simulink library "inp"  (R2021b)
settings: Solver=VariableStepAuto  StartTime=0.0  StopTime=10.0  RelTol=1e-3
undefined symbols (not defined in the file): C_TASK_5MS_S, FALSE, KINP_AcoreReadyToSlp_flg_ovrdflg, KINP_AcoreReadyToSlp_flg_ovrdval, KINP_AllowMovThd_OTA_enum_ovrdflg, KINP_AllowMovThd_OTA_enum_ovrdval, KINP_APSAngleTarget_Deg_ovrdflg, KINP_APSAngleTarget_Deg_ovrdval, KINP_APSDecReq_mps2_ovrdflg, KINP_APSDecReq_mps2_ovrdval, KINP_APSDecReqA_flg_ovrdflg, KINP_APSDecReqA_flg_ovrdval, KINP_APSDFLL_cm_ovrdflg, KINP_APSDFLL_cm_ovrdval, KINP_APSDFLR_cm_ovrdflg, KINP_APSDFLR_cm_ovrdval, KINP_APSDRLL_cm_ovrdflg, KINP_APSDRLL_cm_ovrdval, KINP_APSDRLR_cm_ovrdflg, KINP_APSDRLR_cm_ovrdval, KINP_APSExitCondition_enum_ovrdflg, KINP_APSExitCondition_enum_ovrdval, KINP_APSHWVer_enum_ovrdflg, KINP_APSHWVer_enum_ovrdval, KINP_APSProgressPCT_pct_ovrdflg, KINP_APSProgressPCT_pct_ovrdval, KINP_APSReq_enum_ovrdflg, KINP_APSReq_enum_ovrdval, KINP_APSRQDisplay_enum_ovrdflg, KINP_APSRQDisplay_enum_ovrdval, KINP_APSRqEPASCtrl_flg_ovrdflg, KINP_APSRqEPASCtrl_flg_ovrdval, KINP_APSShiftPosnReq_enum_ovrdval, KINP_APSShiftPosnReq_enum_ovrflg, KINP_APSSpeedCMD_kph_ovrdval, KINP_APSSpeedCMD_kph_ovrflg, KINP_APSStaSystem_enum_ovrdflg, KINP_APSStaSystem_enum_ovrdval, KINP_APSSWVer_enum_ovrdflg, KINP_APSSWVer_enum_ovrdval, KINP_APSVMCReqA_flg_ovrdval, KINP_APSVMCReqA_flg_ovrflg, KINP_APSVRqEPASCtrl_flg_ovrdflg, KINP_APSVRqEPASCtrl_flg_ovrdval, KINP_AuxBattVolmV_mV_ovrdflg, KINP_AuxBattVolmV_mV_ovrdval, KINP_CAASSta_enum_ovrdflg, KINP_CAASSta_enum_ovrdval, KINP_CAASVMCReqA_flg_ovrdval, KINP_CAASVMCReqA_flg_ovrflg, KINP_Chime_enum_ovrdflg, KINP_Chime_enum_ovrdval, KINP_ClearDTCcmd_flg_ovrdflg, KINP_ClearDTCcmd_flg_ovrdval, KINP_EvccAplusPwrUpReq_flg_ovrdflg, KINP_EvccAplusPwrUpReq_flg_ovrdval, KINP_LFID_raw_ovrdval, KINP_LFID_raw_ovrflg, KINP_LRID_raw_ovrdval, KINP_MemOffsetAccX_raw16_ovrdflg ... (+118)
libraries: FVT_lib x942, hcu_lib x1
(part 20 of 31)

== system inp/INP/CAN3/SignalCheck/MCU_B_R1 ==
  BHAL_outputs : Inport
  inp_CanValid_bus : Inport  Port=2
  MCUWarnR : FVT_lib/inp/can_signal_template  SystemSampleTime=-1  VariantActivationTime=update diagram  Latency=0  AutoFrameSizeCalculation=off
      link override defval: Value=KINP_MCUWarnR_enum_defval
      link override ovrdflg: Value=KINP_MCUWarnR_enum_ovrdflg
      link override ovrdval: Value=KINP_MCUWarnR_enum_ovrdval
  RrActvDmpDisabSta : FVT_lib/inp/can_signal_template  SystemSampleTime=-1  VariantActivationTime=update diagram  Latency=0  AutoFrameSizeCalculation=off
      link override defval: Value=KINP_RrActvDmpDisabSta_flg_defval
      link override ovrdflg: Value=KINP_RrActvDmpDisabSta_flg_ovrdflg
      link override ovrdval: Value=KINP_RrActvDmpDisabSta_flg_ovrdval
  RrEDUDrtSta : FVT_lib/inp/can_signal_template  SystemSampleTime=-1  VariantActivationTime=update diagram  Latency=0  AutoFrameSizeCalculation=off
      link override defval: Value=KINP_RrEDUDrtSta_flg_defval
      link override ovrdflg: Value=KINP_RrEDUDrtSta_flg_ovrdflg
      link override ovrdval: Value=KINP_RrEDUDrtSta_flg_ovrdval
  RrEDUOpratingSta : FVT_lib/inp/can_signal_template  SystemSampleTime=-1  VariantActivationTime=update diagram  Latency=0  AutoFrameSizeCalculation=off
      link override defval: Value=KINP_RrEDUOpratingSta_flg_defval
      link override ovrdflg: Value=KINP_RrEDUOpratingSta_flg_ovrdflg
      link override ovrdval: Value=KINP_RrEDUOpratingSta_flg_ovrdval
  RrEDURealTMTq : FVT_lib/inp/can_signal_template  SystemSampleTime=-1  VariantActivationTime=update diagram  Latency=0  AutoFrameSizeCalculation=off
      link override defval: Value=KINP_RrEDURealTMTq_Nm_defval
      link override ovrdflg: Value=KINP_RrEDURealTMTq_Nm_ovrdflg
      link override ovrdval: Value=KINP_RrEDURealTMTq_Nm_ovrdval
  RrEDURotateDirction : FVT_lib/inp/can_signal_template  SystemSampleTime=-1  VariantActivationTime=update diagram  Latency=0  AutoFrameSizeCalculation=off
      link override defval: Value=KINP_RrEDURotateDirction_enum_defval
      link override ovrdflg: Value=KINP_RrEDURotateDirction_enum_ovrdflg
      link override ovrdval: Value=KINP_RrEDURotateDirction_enum_ovrdval
  RrEDUTqReqFbk : FVT_lib/inp/can_signal_template  SystemSampleTime=-1  VariantActivationTime=update diagram  Latency=0  AutoFrameSizeCalculation=off
      link override defval: Value=KINP_RrEDUTqReqFbk_Nm_defval
      link override ovrdflg: Value=KINP_RrEDUTqReqFbk_Nm_ovrdflg
      link override ovrdval: Value=KINP_RrEDUTqReqFbk_Nm_ovrdval
  RrMCUBAT : FVT_lib/inp/can_signal_template  SystemSampleTime=-1  VariantActivationTime=update diagram  Latency=0  AutoFrameSizeCalculation=off
      link override defval: Value=KINP_RrMCUBAT_V_defval
      link override ovrdflg: Value=KINP_RrMCUBAT_V_ovrdflg
      link override ovrdval: Value=KINP_RrMCUBAT_V_ovrdval
  RrMCUDCBusCurr : FVT_lib/inp/can_signal_template  SystemSampleTime=-1  VariantActivationTime=update diagram  Latency=0  AutoFrameSizeCalculation=off
      link override defval: Value=KINP_RrMCUDCBusCurr_A_defval
      link override ovrdflg: Value=KINP_RrMCUDCBusCurr_A_ovrdflg
      link override ovrdval: Value=KINP_RrMCUDCBusCurr_A_ovrdval
  RrMCUDCBusVolt : FVT_lib/inp/can_signal_template  SystemSampleTime=-1  VariantActivationTime=update diagram  Latency=0  AutoFrameSizeCalculation=off
      link override defval: Value=KINP_RrMCUDCBusVolt_V_defval
      link override ovrdflg: Value=KINP_RrMCUDCBusVolt_V_ovrdflg
      link override ovrdval: Value=KINP_RrMCUDCBusVolt_V_ovrdval
  RrMCUDischrgSta : FVT_lib/inp/can_signal_template  SystemSampleTime=-1  VariantActivationTime=update diagram  Latency=0  AutoFrameSizeCalculation=off
      link override defval: Value=KINP_RrMCUDischrgSta_flg_defval
      link override ovrdflg: Value=KINP_RrMCUDischrgSta_flg_ovrdflg
      link override ovrdval: Value=KINP_RrMCUDischrgSta_flg_ovrdval
  RrMCUEnaSta : FVT_lib/inp/can_signal_template  SystemSampleTime=-1  VariantActivationTime=update diagram  Latency=0  AutoFrameSizeCalculation=off
      link override defval: Value=KINP_RrMCUEnaSta_flg_defval
      link override ovrdflg: Value=KINP_RrMCUEnaSta_flg_ovrdflg
      link override ovrdval: Value=KINP_RrMCUEnaSta_flg_ovrdval
  RrMCUErr : FVT_lib/inp/can_signal_template  SystemSampleTime=-1  VariantActivationTime=update diagram  Latency=0  AutoFrameSizeCalculation=off
      link override defval: Value=KINP_RrMCUErr_enum_defval
      link override ovrdflg: Value=KINP_RrMCUErr_enum_ovrdflg
      link override ovrdval: Value=KINP_RrMCUErr_enum_ovrdval
  RrMCUIGNsta : FVT_lib/inp/can_signal_template  SystemSampleTime=-1  VariantActivationTime=update diagram  Latency=0  AutoFrameSizeCalculation=off
      link override defval: Value=KINP_RrMCUIGNsta_flg_defval
      link override ovrdflg: Value=KINP_RrMCUIGNsta_flg_ovrdflg
      link override ovrdval: Value=KINP_RrMCUIGNsta_flg_ovrdval
  RrMCUReady : FVT_lib/inp/can_signal_template  SystemSampleTime=-1  VariantActivationTime=update diagram  Latency=0  AutoFrameSizeCalculation=off
      link override defval: Value=KINP_RrMCUReady_flg_defval
      link override ovrdflg: Value=KINP_RrMCUReady_flg_ovrdflg
      link override ovrdval: Value=KINP_RrMCUReady_flg_ovrdval
  RrMCUReady4Pre : FVT_lib/inp/can_signal_template  SystemSampleTime=-1  VariantActivationTime=update diagram  Latency=0  AutoFrameSizeCalculation=off
      link override defval: Value=KINP_RrMCUReady4Pre_flg_defval
      link override ovrdflg: Value=KINP_RrMCUReady4Pre_flg_ovrdflg
      link override ovrdval: Value=KINP_RrMCUReady4Pre_flg_ovrdval
  RrMCUSysSta : FVT_lib/inp/can_signal_template  SystemSampleTime=-1  VariantActivationTime=update diagram  Latency=0  AutoFrameSizeCalculation=off
      link override defval: Value=KINP_RrMCUSysSta_enum_defval
      link override ovrdflg: Value=KINP_RrMCUSysSta_enum_ovrdflg
      link override ovrdval: Value=KINP_RrMCUSysSta_enum_ovrdval
  RrMCUTemp : FVT_lib/inp/can_signal_template  SystemSampleTime=-1  VariantActivationTime=update diagram  Latency=0  AutoFrameSizeCalculation=off
      link override defval: Value=KINP_RrMCUTemp_C_defval
      link override ovrdflg: Value=KINP_RrMCUTemp_C_ovrdflg
      link override ovrdval: Value=KINP_RrMCUTemp_C_ovrdval
  RrMotorAvailTq : FVT_lib/inp/can_signal_template  SystemSampleTime=-1  VariantActivationTime=update diagram  Latency=0  AutoFrameSizeCalculation=off
      link override defval: Value=KINP_RrMotorAvailTq_Nm_defval
      link override ovrdflg: Value=KINP_RrMotorAvailTq_Nm_ovrdflg
      link override ovrdval: Value=KINP_RrMotorAvailTq_Nm_ovrdval
  RrRegenAvailTq : FVT_lib/inp/can_signal_template  SystemSampleTime=-1  VariantActivationTime=update diagram  Latency=0  AutoFrameSizeCalculation=off
      link override defval: Value=KINP_RrRegenAvailTq_Nm_defval
      link override ovrdflg: Value=KINP_RrRegenAvailTq_Nm_ovrdflg
      link override ovrdval: Value=KINP_RrRegenAvailTq_Nm_ovrdval
  RrTMSpd : FVT_lib/inp/can_signal_template  SystemSampleTime=-1  VariantActivationTime=update diagram  Latency=0  AutoFrameSizeCalculation=off
      link override defval: Value=KINP_RrTMSpd_rpm_defval
      link override ovrdflg: Value=KINP_RrTMSpd_rpm_ovrdflg
      link override ovrdval: Value=KINP_RrTMSpd_rpm_ovrdval
  RrTMTemp : FVT_lib/inp/can_signal_template  SystemSampleTime=-1  VariantActivationTime=update diagram  Latency=0  AutoFrameSizeCalculation=off
      link override defval: Value=KINP_RrTMTemp_C_defval
      link override ovrdflg: Value=KINP_RrTMTemp_C_ovrdflg
      link override ovrdval: Value=KINP_RrTMTemp_C_ovrdval
  RrTMid : FVT_lib/inp/can_signal_template  SystemSampleTime=-1  VariantActivationTime=update diagram  Latency=0  AutoFrameSizeCalculation=off
      link override defval: Value=KINP_RrTMid_A_defval
      link override ovrdflg: Value=KINP_RrTMid_A_ovrdflg
      link override ovrdval: Value=KINP_RrTMid_A_ovrdval
  RrTMiq : FVT_lib/inp/can_signal_template  SystemSampleTime=-1  VariantActivationTime=update diagram  Latency=0  AutoFrameSizeCalculation=off
      link override defval: Value=KINP_RrTMiq_A_defval
      link override ovrdflg: Value=KINP_RrTMiq_A_ovrdflg
      link override ovrdval: Value=KINP_RrTMiq_A_ovrdval
  Terminator_{1..24} (24 alike) : Terminator
  True_VHAL_MCUWarnR_enum : Constant  Value=TRUE  OutDataTypeStr=boolean
  True_VHAL_RrActvDmpDisabSta_flg : Constant  Value=TRUE  OutDataTypeStr=boolean
  True_VHAL_RrEDUDrtSta_flg : Constant  Value=TRUE  OutDataTypeStr=boolean
  True_VHAL_RrEDUOpratingSta_flg : Constant  Value=TRUE  OutDataTypeStr=boolean
  True_VHAL_RrEDURealTMTq_Nm : Constant  Value=TRUE  OutDataTypeStr=boolean
  True_VHAL_RrEDURotateDirction_enum : Constant  Value=TRUE  OutDataTypeStr=boolean
  True_VHAL_RrEDUTqReqFbk_Nm : Constant  Value=TRUE  OutDataTypeStr=boolean
  True_VHAL_RrMCUBAT_V : Constant  Value=TRUE  OutDataTypeStr=boolean
  True_VHAL_RrMCUDCBusCurr_A : Constant  Value=TRUE  OutDataTypeStr=boolean
  True_VHAL_RrMCUDCBusVolt_V : Constant  Value=TRUE  OutDataTypeStr=boolean
  True_VHAL_RrMCUDischrgSta_flg : Constant  Value=TRUE  OutDataTypeStr=boolean
  True_VHAL_RrMCUEnaSta_flg : Constant  Value=TRUE  OutDataTypeStr=boolean
  True_VHAL_RrMCUErr_enum : Constant  Value=TRUE  OutDataTypeStr=boolean
  True_VHAL_RrMCUIGNsta_flg : Constant  Value=TRUE  OutDataTypeStr=boolean
  True_VHAL_RrMCUReady4Pre_flg : Constant  Value=TRUE  OutDataTypeStr=boolean
  True_VHAL_RrMCUReady_flg : Constant  Value=TRUE  OutDataTypeStr=boolean
  True_VHAL_RrMCUSysSta_enum : Constant  Value=TRUE  OutDataTypeStr=boolean
  True_VHAL_RrMCUTemp_C : Constant  Value=TRUE  OutDataTypeStr=boolean
  True_VHAL_RrMotorAvailTq_Nm : Constant  Value=TRUE  OutDataTypeStr=boolean
  True_VHAL_RrRegenAvailTq_Nm : Constant  Value=TRUE  OutDataTypeStr=boolean
  True_VHAL_RrTMSpd_rpm : Constant  Value=TRUE  OutDataTypeStr=boolean
  True_VHAL_RrTMTemp_C : Constant  Value=TRUE  OutDataTypeStr=boolean
  True_VHAL_RrTMid_A : Constant  Value=TRUE  OutDataTypeStr=boolean
  True_VHAL_RrTMiq_A : Constant  Value=TRUE  OutDataTypeStr=boolean
  slr1_{1..24} (24 alike) : BusSelector  OutputSignals=VINP_CANMsgValidMCUBR1_flg
  slr_VHAL_MCUWarnR_enum : BusSelector  OutputSignals=VHAL_MCUWarnR_enum
  slr_VHAL_RrActvDmpDisabSta_flg : BusSelector  OutputSignals=VHAL_RrActvDmpDisabSta_flg
  slr_VHAL_RrEDUDrtSta_flg : BusSelector  OutputSignals=VHAL_RrEDUDrtSta_flg
  slr_VHAL_RrEDUOpratingSta_flg : BusSelector  OutputSignals=VHAL_RrEDUOpratingSta_flg
  slr_VHAL_RrEDURealTMTq_Nm : BusSelector  OutputSignals=VHAL_RrEDURealTMTq_Nm
  slr_VHAL_RrEDURotateDirction_enum : BusSelector  OutputSignals=VHAL_RrEDURotateDirction_enum
  slr_VHAL_RrEDUTqReqFbk_Nm : BusSelector  OutputSignals=VHAL_RrEDUTqReqFbk_Nm
  slr_VHAL_RrMCUBAT_V : BusSelector  OutputSignals=VHAL_RrMCUBAT_V
  slr_VHAL_RrMCUDCBusCurr_A : BusSelector  OutputSignals=VHAL_RrMCUDCBusCurr_A
  slr_VHAL_RrMCUDCBusVolt_V : BusSelector  OutputSignals=VHAL_RrMCUDCBusVolt_V
  slr_VHAL_RrMCUDischrgSta_flg : BusSelector  OutputSignals=VHAL_RrMCUDischrgSta_flg
  slr_VHAL_RrMCUEnaSta_flg : BusSelector  OutputSignals=VHAL_RrMCUEnaSta_flg
  slr_VHAL_RrMCUErr_enum : BusSelector  OutputSignals=VHAL_RrMCUErr_enum
  slr_VHAL_RrMCUIGNsta_flg : BusSelector  OutputSignals=VHAL_RrMCUIGNsta_flg
  slr_VHAL_RrMCUReady4Pre_flg : BusSelector  OutputSignals=VHAL_RrMCUReady4Pre_flg
  slr_VHAL_RrMCUReady_flg : BusSelector  OutputSignals=VHAL_RrMCUReady_flg
  slr_VHAL_RrMCUSysSta_enum : BusSelector  OutputSignals=VHAL_RrMCUSysSta_enum
  slr_VHAL_RrMCUTemp_C : BusSelector  OutputSignals=VHAL_RrMCUTemp_C
  slr_VHAL_RrMotorAvailTq_Nm : BusSelector  OutputSignals=VHAL_RrMotorAvailTq_Nm
  slr_VHAL_RrRegenAvailTq_Nm : BusSelector  OutputSignals=VHAL_RrRegenAvailTq_Nm
  slr_VHAL_RrTMSpd_rpm : BusSelector  OutputSignals=VHAL_RrTMSpd_rpm
  slr_VHAL_RrTMTemp_C : BusSelector  OutputSignals=VHAL_RrTMTemp_C
  slr_VHAL_RrTMid_A : BusSelector  OutputSignals=VHAL_RrTMid_A
  slr_VHAL_RrTMiq_A : BusSelector  OutputSignals=VHAL_RrTMiq_A
  VINP_MCUWarnR_enum : Outport
  VINP_RrActvDmpDisabSta_flg : Outport  Port=2
  VINP_RrEDUDrtSta_flg : Outport  Port=3
  VINP_RrEDUOpratingSta_flg : Outport  Port=4
  VINP_RrEDURealTMTq_Nm : Outport  Port=5
  VINP_RrEDURotateDirction_enum : Outport  Port=6
  VINP_RrEDUTqReqFbk_Nm : Outport  Port=7
  VINP_RrMCUBAT_V : Outport  Port=8
  VINP_RrMCUDCBusCurr_A : Outport  Port=9
  VINP_RrMCUDCBusVolt_V : Outport  Port=10
  VINP_RrMCUDischrgSta_flg : Outport  Port=11
  VINP_RrMCUEnaSta_flg : Outport  Port=12
  VINP_RrMCUErr_enum : Outport  Port=13
  VINP_RrMCUIGNsta_flg : Outport  Port=14
  VINP_RrMCUReady_flg : Outport  Port=15
  VINP_RrMCUReady4Pre_flg : Outport  Port=16
  VINP_RrMCUSysSta_enum : Outport  Port=17
  VINP_RrMCUTemp_C : Outport  Port=18
  VINP_RrMotorAvailTq_Nm : Outport  Port=19
  VINP_RrRegenAvailTq_Nm : Outport  Port=20
  VINP_RrTMSpd_rpm : Outport  Port=21
  VINP_RrTMTemp_C : Outport  Port=22
  VINP_RrTMid_A : Outport  Port=23
  VINP_RrTMiq_A : Outport  Port=24
  wires:
  BHAL_outputs/1 -> [BHAL_outputs]
  inp_CanValid_bus/1 -> [inp_CanValid_bus]
  [BHAL_outputs] -> slr_VHAL_MCUWarnR_enum/1
  slr_VHAL_MCUWarnR_enum/1 -> MCUWarnR/1  "<VHAL_MCUWarnR_enum>"
  True_VHAL_MCUWarnR_enum/1 -> MCUWarnR/2
  [inp_CanValid_bus] -> slr1_1/1
  slr1_1/1 -> MCUWarnR/3  "<VINP_CANMsgValidMCUBR1_flg>"
  MCUWarnR/1 -> VINP_MCUWarnR_enum/1  "VINP_MCUWarnR_enum"
  MCUWarnR/2 -> Terminator_1/1
  [BHAL_outputs] -> slr_VHAL_RrActvDmpDisabSta_flg/1
  slr_VHAL_RrActvDmpDisabSta_flg/1 -> RrActvDmpDisabSta/1  "<VHAL_RrActvDmpDisabSta_flg>"
  True_VHAL_RrActvDmpDisabSta_flg/1 -> RrActvDmpDisabSta/2
  [inp_CanValid_bus] -> slr1_2/1
  slr1_2/1 -> RrActvDmpDisabSta/3  "<VINP_CANMsgValidMCUBR1_flg>"
  RrActvDmpDisabSta/1 -> VINP_RrActvDmpDisabSta_flg/1  "VINP_RrActvDmpDisabSta_flg"
  RrActvDmpDisabSta/2 -> Terminator_2/1
  [BHAL_outputs] -> slr_VHAL_RrEDUDrtSta_flg/1
  slr_VHAL_RrEDUDrtSta_flg/1 -> RrEDUDrtSta/1  "<VHAL_RrEDUDrtSta_flg>"
  True_VHAL_RrEDUDrtSta_flg/1 -> RrEDUDrtSta/2
  [inp_CanValid_bus] -> slr1_3/1
  slr1_3/1 -> RrEDUDrtSta/3  "<VINP_CANMsgValidMCUBR1_flg>"
  RrEDUDrtSta/1 -> VINP_RrEDUDrtSta_flg/1  "VINP_RrEDUDrtSta_flg"
  RrEDUDrtSta/2 -> Terminator_3/1
  [BHAL_outputs] -> slr_VHAL_RrEDUOpratingSta_flg/1
  slr_VHAL_RrEDUOpratingSta_flg/1 -> RrEDUOpratingSta/1  "<VHAL_RrEDUOpratingSta_flg>"
  True_VHAL_RrEDUOpratingSta_flg/1 -> RrEDUOpratingSta/2
  [inp_CanValid_bus] -> slr1_4/1
  slr1_4/1 -> RrEDUOpratingSta/3  "<VINP_CANMsgValidMCUBR1_flg>"
  RrEDUOpratingSta/1 -> VINP_RrEDUOpratingSta_flg/1  "VINP_RrEDUOpratingSta_flg"
  RrEDUOpratingSta/2 -> Terminator_4/1
  [BHAL_outputs] -> slr_VHAL_RrEDURealTMTq_Nm/1
  slr_VHAL_RrEDURealTMTq_Nm/1 -> RrEDURealTMTq/1  "<VHAL_RrEDURealTMTq_Nm>"
  True_VHAL_RrEDURealTMTq_Nm/1 -> RrEDURealTMTq/2
  [inp_CanValid_bus] -> slr1_5/1
  slr1_5/1 -> RrEDURealTMTq/3  "<VINP_CANMsgValidMCUBR1_flg>"
  RrEDURealTMTq/1 -> VINP_RrEDURealTMTq_Nm/1  "VINP_RrEDURealTMTq_Nm"
  RrEDURealTMTq/2 -> Terminator_5/1
  [BHAL_outputs] -> slr_VHAL_RrEDURotateDirction_enum/1
  slr_VHAL_RrEDURotateDirction_enum/1 -> RrEDURotateDirction/1  "<VHAL_RrEDURotateDirction_enum>"
  True_VHAL_RrEDURotateDirction_enum/1 -> RrEDURotateDirction/2
  [inp_CanValid_bus] -> slr1_6/1
  slr1_6/1 -> RrEDURotateDirction/3  "<VINP_CANMsgValidMCUBR1_flg>"
  RrEDURotateDirction/1 -> VINP_RrEDURotateDirction_enum/1  "VINP_RrEDURotateDirction_enum"
  RrEDURotateDirction/2 -> Terminator_6/1
  [BHAL_outputs] -> slr_VHAL_RrEDUTqReqFbk_Nm/1
  slr_VHAL_RrEDUTqReqFbk_Nm/1 -> RrEDUTqReqFbk/1  "<VHAL_RrEDUTqReqFbk_Nm>"
  True_VHAL_RrEDUTqReqFbk_Nm/1 -> RrEDUTqReqFbk/2
  [inp_CanValid_bus] -> slr1_7/1
  slr1_7/1 -> RrEDUTqReqFbk/3  "<VINP_CANMsgValidMCUBR1_flg>"
  RrEDUTqReqFbk/1 -> VINP_RrEDUTqReqFbk_Nm/1  "VINP_RrEDUTqReqFbk_Nm"
  RrEDUTqReqFbk/2 -> Terminator_7/1
  [BHAL_outputs] -> slr_VHAL_RrMCUBAT_V/1
  slr_VHAL_RrMCUBAT_V/1 -> RrMCUBAT/1  "<VHAL_RrMCUBAT_V>"
  True_VHAL_RrMCUBAT_V/1 -> RrMCUBAT/2
  [inp_CanValid_bus] -> slr1_8/1
  slr1_8/1 -> RrMCUBAT/3  "<VINP_CANMsgValidMCUBR1_flg>"
  RrMCUBAT/1 -> VINP_RrMCUBAT_V/1  "VINP_RrMCUBAT_V"
  RrMCUBAT/2 -> Terminator_8/1
  [BHAL_outputs] -> slr_VHAL_RrMCUDCBusCurr_A/1
  slr_VHAL_RrMCUDCBusCurr_A/1 -> RrMCUDCBusCurr/1  "<VHAL_RrMCUDCBusCurr_A>"
  True_VHAL_RrMCUDCBusCurr_A/1 -> RrMCUDCBusCurr/2
  [inp_CanValid_bus] -> slr1_9/1
  slr1_9/1 -> RrMCUDCBusCurr/3  "<VINP_CANMsgValidMCUBR1_flg>"
  RrMCUDCBusCurr/1 -> VINP_RrMCUDCBusCurr_A/1  "VINP_RrMCUDCBusCurr_A"
  RrMCUDCBusCurr/2 -> Terminator_9/1
  [BHAL_outputs] -> slr_VHAL_RrMCUDCBusVolt_V/1
  slr_VHAL_RrMCUDCBusVolt_V/1 -> RrMCUDCBusVolt/1  "<VHAL_RrMCUDCBusVolt_V>"
  True_VHAL_RrMCUDCBusVolt_V/1 -> RrMCUDCBusVolt/2
  [inp_CanValid_bus] -> slr1_10/1
  slr1_10/1 -> RrMCUDCBusVolt/3  "<VINP_CANMsgValidMCUBR1_flg>"
  RrMCUDCBusVolt/1 -> VINP_RrMCUDCBusVolt_V/1  "VINP_RrMCUDCBusVolt_V"
  RrMCUDCBusVolt/2 -> Terminator_10/1
  [BHAL_outputs] -> slr_VHAL_RrMCUDischrgSta_flg/1
  slr_VHAL_RrMCUDischrgSta_flg/1 -> RrMCUDischrgSta/1  "<VHAL_RrMCUDischrgSta_flg>"
  True_VHAL_RrMCUDischrgSta_flg/1 -> RrMCUDischrgSta/2
  [inp_CanValid_bus] -> slr1_11/1
  slr1_11/1 -> RrMCUDischrgSta/3  "<VINP_CANMsgValidMCUBR1_flg>"
  RrMCUDischrgSta/1 -> VINP_RrMCUDischrgSta_flg/1  "VINP_RrMCUDischrgSta_flg"
  RrMCUDischrgSta/2 -> Terminator_11/1
  [BHAL_outputs] -> slr_VHAL_RrMCUEnaSta_flg/1
  slr_VHAL_RrMCUEnaSta_flg/1 -> RrMCUEnaSta/1  "<VHAL_RrMCUEnaSta_flg>"
  True_VHAL_RrMCUEnaSta_flg/1 -> RrMCUEnaSta/2
  [inp_CanValid_bus] -> slr1_12/1
  slr1_12/1 -> RrMCUEnaSta/3  "<VINP_CANMsgValidMCUBR1_flg>"
  RrMCUEnaSta/1 -> VINP_RrMCUEnaSta_flg/1  "VINP_RrMCUEnaSta_flg"
  RrMCUEnaSta/2 -> Terminator_12/1
  [BHAL_outputs] -> slr_VHAL_RrMCUErr_enum/1
  slr_VHAL_RrMCUErr_enum/1 -> RrMCUErr/1  "<VHAL_RrMCUErr_enum>"
  True_VHAL_RrMCUErr_enum/1 -> RrMCUErr/2
  [inp_CanValid_bus] -> slr1_13/1
  slr1_13/1 -> RrMCUErr/3  "<VINP_CANMsgValidMCUBR1_flg>"
  RrMCUErr/1 -> VINP_RrMCUErr_enum/1  "VINP_RrMCUErr_enum"
  RrMCUErr/2 -> Terminator_13/1
  [BHAL_outputs] -> slr_VHAL_RrMCUIGNsta_flg/1
  slr_VHAL_RrMCUIGNsta_flg/1 -> RrMCUIGNsta/1  "<VHAL_RrMCUIGNsta_flg>"
  True_VHAL_RrMCUIGNsta_flg/1 -> RrMCUIGNsta/2
  [inp_CanValid_bus] -> slr1_14/1
  slr1_14/1 -> RrMCUIGNsta/3  "<VINP_CANMsgValidMCUBR1_flg>"
  RrMCUIGNsta/1 -> VINP_RrMCUIGNsta_flg/1  "VINP_RrMCUIGNsta_flg"
  RrMCUIGNsta/2 -> Terminator_14/1
  [BHAL_outputs] -> slr_VHAL_RrMCUReady_flg/1
  slr_VHAL_RrMCUReady_flg/1 -> RrMCUReady/1  "<VHAL_RrMCUReady_flg>"
  True_VHAL_RrMCUReady_flg/1 -> RrMCUReady/2
  [inp_CanValid_bus] -> slr1_15/1
  slr1_15/1 -> RrMCUReady/3  "<VINP_CANMsgValidMCUBR1_flg>"
  RrMCUReady/1 -> VINP_RrMCUReady_flg/1  "VINP_RrMCUReady_flg"
  RrMCUReady/2 -> Terminator_15/1
  [BHAL_outputs] -> slr_VHAL_RrMCUReady4Pre_flg/1
  slr_VHAL_RrMCUReady4Pre_flg/1 -> RrMCUReady4Pre/1  "<VHAL_RrMCUReady4Pre_flg>"
  True_VHAL_RrMCUReady4Pre_flg/1 -> RrMCUReady4Pre/2
  [inp_CanValid_bus] -> slr1_16/1
  slr1_16/1 -> RrMCUReady4Pre/3  "<VINP_CANMsgValidMCUBR1_flg>"
  RrMCUReady4Pre/1 -> VINP_RrMCUReady4Pre_flg/1  "VINP_RrMCUReady4Pre_flg"
  RrMCUReady4Pre/2 -> Terminator_16/1
  [BHAL_outputs] -> slr_VHAL_RrMCUSysSta_enum/1
  slr_VHAL_RrMCUSysSta_enum/1 -> RrMCUSysSta/1  "<VHAL_RrMCUSysSta_enum>"
  True_VHAL_RrMCUSysSta_enum/1 -> RrMCUSysSta/2
  [inp_CanValid_bus] -> slr1_17/1
  slr1_17/1 -> RrMCUSysSta/3  "<VINP_CANMsgValidMCUBR1_flg>"
  RrMCUSysSta/1 -> VINP_RrMCUSysSta_enum/1  "VINP_RrMCUSysSta_enum"
  RrMCUSysSta/2 -> Terminator_17/1
  [BHAL_outputs] -> slr_VHAL_RrMCUTemp_C/1
  slr_VHAL_RrMCUTemp_C/1 -> RrMCUTemp/1  "<VHAL_RrMCUTemp_C>"
  True_VHAL_RrMCUTemp_C/1 -> RrMCUTemp/2
  [inp_CanValid_bus] -> slr1_18/1
  slr1_18/1 -> RrMCUTemp/3  "<VINP_CANMsgValidMCUBR1_flg>"
  RrMCUTemp/1 -> VINP_RrMCUTemp_C/1  "VINP_RrMCUTemp_C"
  RrMCUTemp/2 -> Terminator_18/1
  [BHAL_outputs] -> slr_VHAL_RrMotorAvailTq_Nm/1
  slr_VHAL_RrMotorAvailTq_Nm/1 -> RrMotorAvailTq/1  "<VHAL_RrMotorAvailTq_Nm>"
  True_VHAL_RrMotorAvailTq_Nm/1 -> RrMotorAvailTq/2
  [inp_CanValid_bus] -> slr1_19/1
  slr1_19/1 -> RrMotorAvailTq/3  "<VINP_CANMsgValidMCUBR1_flg>"
  RrMotorAvailTq/1 -> VINP_RrMotorAvailTq_Nm/1  "VINP_RrMotorAvailTq_Nm"
  RrMotorAvailTq/2 -> Terminator_19/1
  [BHAL_outputs] -> slr_VHAL_RrRegenAvailTq_Nm/1
  slr_VHAL_RrRegenAvailTq_Nm/1 -> RrRegenAvailTq/1  "<VHAL_RrRegenAvailTq_Nm>"
  True_VHAL_RrRegenAvailTq_Nm/1 -> RrRegenAvailTq/2
  [inp_CanValid_bus] -> slr1_20/1
  slr1_20/1 -> RrRegenAvailTq/3  "<VINP_CANMsgValidMCUBR1_flg>"
  RrRegenAvailTq/1 -> VINP_RrRegenAvailTq_Nm/1  "VINP_RrRegenAvailTq_Nm"
  RrRegenAvailTq/2 -> Terminator_20/1
  [BHAL_outputs] -> slr_VHAL_RrTMSpd_rpm/1
  slr_VHAL_RrTMSpd_rpm/1 -> RrTMSpd/1  "<VHAL_RrTMSpd_rpm>"
  True_VHAL_RrTMSpd_rpm/1 -> RrTMSpd/2
  [inp_CanValid_bus] -> slr1_21/1
  slr1_21/1 -> RrTMSpd/3  "<VINP_CANMsgValidMCUBR1_flg>"
  RrTMSpd/1 -> VINP_RrTMSpd_rpm/1  "VINP_RrTMSpd_rpm"
  RrTMSpd/2 -> Terminator_21/1
  [BHAL_outputs] -> slr_VHAL_RrTMTemp_C/1
  slr_VHAL_RrTMTemp_C/1 -> RrTMTemp/1  "<VHAL_RrTMTemp_C>"
  True_VHAL_RrTMTemp_C/1 -> RrTMTemp/2
  [inp_CanValid_bus] -> slr1_22/1
  slr1_22/1 -> RrTMTemp/3  "<VINP_CANMsgValidMCUBR1_flg>"
  RrTMTemp/1 -> VINP_RrTMTemp_C/1  "VINP_RrTMTemp_C"
  RrTMTemp/2 -> Terminator_22/1
  [BHAL_outputs] -> slr_VHAL_RrTMid_A/1
  slr_VHAL_RrTMid_A/1 -> RrTMid/1  "<VHAL_RrTMid_A>"
  True_VHAL_RrTMid_A/1 -> RrTMid/2
  [inp_CanValid_bus] -> slr1_23/1
  slr1_23/1 -> RrTMid/3  "<VINP_CANMsgValidMCUBR1_flg>"
  RrTMid/1 -> VINP_RrTMid_A/1  "VINP_RrTMid_A"
  RrTMid/2 -> Terminator_23/1
  [BHAL_outputs] -> slr_VHAL_RrTMiq_A/1
  slr_VHAL_RrTMiq_A/1 -> RrTMiq/1  "<VHAL_RrTMiq_A>"
  True_VHAL_RrTMiq_A/1 -> RrTMiq/2
  [inp_CanValid_bus] -> slr1_24/1
  slr1_24/1 -> RrTMiq/3  "<VINP_CANMsgValidMCUBR1_flg>"
  RrTMiq/1 -> VINP_RrTMiq_A/1  "VINP_RrTMiq_A"
  RrTMiq/2 -> Terminator_24/1

== system inp/INP/CAN3/SignalCheck/MCU_B_R2 ==
  BHAL_outputs : Inport
  inp_CanValid_bus : Inport  Port=2
  MCUBRLLCTempWarnSta : FVT_lib/inp/can_signal_template  SystemSampleTime=-1  VariantActivationTime=update diagram  Latency=0  AutoFrameSizeCalculation=off
      link override defval: Value=KINP_MCUBRLLCTempWarnSta_enum_defval
      link override ovrdflg: Value=KINP_MCUBRLLCTempWarnSta_enum_ovrdflg
      link override ovrdval: Value=KINP_MCUBRLLCTempWarnSta_enum_ovrdval
  RrCoolanttempReq : FVT_lib/inp/can_signal_template  SystemSampleTime=-1  VariantActivationTime=update diagram  Latency=0  AutoFrameSizeCalculation=off
      link override defval: Value=KINP_RrCoolanttempReq_cnt_defval
      link override ovrdflg: Value=KINP_RrCoolanttempReq_cnt_ovrdflg
      link override ovrdval: Value=KINP_RrCoolanttempReq_cnt_ovrdval
  RrFailcode1 : FVT_lib/inp/can_signal_template  SystemSampleTime=-1  VariantActivationTime=update diagram  Latency=0  AutoFrameSizeCalculation=off
      link override defval: Value=KINP_RrFailcode1_enum_defval
      link override ovrdflg: Value=KINP_RrFailcode1_enum_ovrdflg
      link override ovrdval: Value=KINP_RrFailcode1_enum_ovrdval
  RrFailcode2 : FVT_lib/inp/can_signal_template  SystemSampleTime=-1  VariantActivationTime=update diagram  Latency=0  AutoFrameSizeCalculation=off
      link override defval: Value=KINP_RrFailcode2_enum_defval
      link override ovrdflg: Value=KINP_RrFailcode2_enum_ovrdflg
      link override ovrdval: Value=KINP_RrFailcode2_enum_ovrdval
  RrFailcodehistory1 : FVT_lib/inp/can_signal_template  SystemSampleTime=-1  VariantActivationTime=update diagram  Latency=0  AutoFrameSizeCalculation=off
      link override defval: Value=KINP_RrFailcodehistory1_enum_defval
      link override ovrdflg: Value=KINP_RrFailcodehistory1_enum_ovrdflg
      link override ovrdval: Value=KINP_RrFailcodehistory1_enum_ovrdval
  RrFailcodehistory2 : FVT_lib/inp/can_signal_template  SystemSampleTime=-1  VariantActivationTime=update diagram  Latency=0  AutoFrameSizeCalculation=off
      link override defval: Value=KINP_RrFailcodehistory2_enum_defval
      link override ovrdflg: Value=KINP_RrFailcodehistory2_enum_ovrdflg
      link override ovrdval: Value=KINP_RrFailcodehistory2_enum_ovrdval
  RrLLCTemp : FVT_lib/inp/can_signal_template  SystemSampleTime=-1  VariantActivationTime=update diagram  Latency=0  AutoFrameSizeCalculation=off
      link override defval: Value=KINP_RrLLCTemp_C_defval
      link override ovrdflg: Value=KINP_RrLLCTemp_C_ovrdflg
      link override ovrdval: Value=KINP_RrLLCTemp_C_ovrdval
  RrLLCflowReq : FVT_lib/inp/can_signal_template  SystemSampleTime=-1  VariantActivationTime=update diagram  Latency=0  AutoFrameSizeCalculation=off
      link override defval: Value=KINP_RrLLCflowReq_Lpmin_defval
      link override ovrdflg: Value=KINP_RrLLCflowReq_Lpmin_ovrdflg
      link override ovrdval: Value=KINP_RrLLCflowReq_Lpmin_ovrdval
  RrMCU3HWVer : FVT_lib/inp/can_signal_template  SystemSampleTime=-1  VariantActivationTime=update diagram  Latency=0  AutoFrameSizeCalculation=off
      link override defval: Value=KINP_RrMCU3HWVer_enum_defval
      link override ovrdflg: Value=KINP_RrMCU3HWVer_enum_ovrdflg
      link override ovrdval: Value=KINP_RrMCU3HWVer_enum_ovrdval
  RrMCU3SWVer : FVT_lib/inp/can_signal_template  SystemSampleTime=-1  VariantActivationTime=update diagram  Latency=0  AutoFrameSizeCalculation=off
      link override defval: Value=KINP_RrMCU3SWVer_enum_defval
      link override ovrdflg: Value=KINP_RrMCU3SWVer_enum_ovrdflg
      link override ovrdval: Value=KINP_RrMCU3SWVer_enum_ovrdval
  RrMCUTempWarn : FVT_lib/inp/can_signal_template  SystemSampleTime=-1  VariantActivationTime=update diagram  Latency=0  AutoFrameSizeCalculation=off
      link override defval: Value=KINP_RrMCUTempWarn_enum_defval
      link override ovrdflg: Value=KINP_RrMCUTempWarn_enum_ovrdflg
      link override ovrdval: Value=KINP_RrMCUTempWarn_enum_ovrdval
  RrTMTempWarn : FVT_lib/inp/can_signal_template  SystemSampleTime=-1  VariantActivationTime=update diagram  Latency=0  AutoFrameSizeCalculation=off
      link override defval: Value=KINP_RrTMTempWarn_enum_defval
      link override ovrdflg: Value=KINP_RrTMTempWarn_enum_ovrdflg
      link override ovrdval: Value=KINP_RrTMTempWarn_enum_ovrdval
  Terminator_{1..12} (12 alike) : Terminator
  True_VHAL_MCUBRLLCTempWarnSta_enum : Constant  Value=TRUE  OutDataTypeStr=boolean
  True_VHAL_RrCoolanttempReq_cnt : Constant  Value=TRUE  OutDataTypeStr=boolean
  True_VHAL_RrFailcode1_enum : Constant  Value=TRUE  OutDataTypeStr=boolean
  True_VHAL_RrFailcode2_enum : Constant  Value=TRUE  OutDataTypeStr=boolean
  True_VHAL_RrFailcodehistory1_enum : Constant  Value=TRUE  OutDataTypeStr=boolean
  True_VHAL_RrFailcodehistory2_enum : Constant  Value=TRUE  OutDataTypeStr=boolean
  True_VHAL_RrLLCTemp_C : Constant  Value=TRUE  OutDataTypeStr=boolean
  True_VHAL_RrLLCflowReq_Lpmin : Constant  Value=TRUE  OutDataTypeStr=boolean
  True_VHAL_RrMCU3HWVer_enum : Constant  Value=TRUE  OutDataTypeStr=boolean
  True_VHAL_RrMCU3SWVer_enum : Constant  Value=TRUE  OutDataTypeStr=boolean
  True_VHAL_RrMCUTempWarn_enum : Constant  Value=TRUE  OutDataTypeStr=boolean
  True_VHAL_RrTMTempWarn_enum : Constant  Value=TRUE  OutDataTypeStr=boolean
  slr1_{1..12} (12 alike) : BusSelector  OutputSignals=VINP_CANMsgValidMCUBR2_flg
  slr_VHAL_MCUBRLLCTempWarnSta_enum : BusSelector  OutputSignals=VHAL_MCUBRLLCTempWarnSta_enum
  slr_VHAL_RrCoolanttempReq_cnt : BusSelector  OutputSignals=VHAL_RrCoolanttempReq_cnt
  slr_VHAL_RrFailcode1_enum : BusSelector  OutputSignals=VHAL_RrFailcode1_enum
  slr_VHAL_RrFailcode2_enum : BusSelector  OutputSignals=VHAL_RrFailcode2_enum
  slr_VHAL_RrFailcodehistory1_enum : BusSelector  OutputSignals=VHAL_RrFailcodehistory1_enum
  slr_VHAL_RrFailcodehistory2_enum : BusSelector  OutputSignals=VHAL_RrFailcodehistory2_enum
  slr_VHAL_RrLLCTemp_C : BusSelector  OutputSignals=VHAL_RrLLCTemp_C
  slr_VHAL_RrLLCflowReq_Lpmin : BusSelector  OutputSignals=VHAL_RrLLCflowReq_Lpmin
  slr_VHAL_RrMCU3HWVer_enum : BusSelector  OutputSignals=VHAL_RrMCU3HWVer_enum
  slr_VHAL_RrMCU3SWVer_enum : BusSelector  OutputSignals=VHAL_RrMCU3SWVer_enum
  slr_VHAL_RrMCUTempWarn_enum : BusSelector  OutputSignals=VHAL_RrMCUTempWarn_enum
  slr_VHAL_RrTMTempWarn_enum : BusSelector  OutputSignals=VHAL_RrTMTempWarn_enum
  VINP_MCUBRLLCTempWarnSta_enum : Outport
  VINP_RrCoolanttempReq_cnt : Outport  Port=2
  VINP_RrFailcode1_enum : Outport  Port=3
  VINP_RrFailcode2_enum : Outport  Port=4
  VINP_RrFailcodehistory1_enum : Outport  Port=5
  VINP_RrFailcodehistory2_enum : Outport  Port=6
  VINP_RrLLCTemp_C : Outport  Port=7
  VINP_RrLLCflowReq_Lpmin : Outport  Port=8
  VINP_RrMCU3HWVer_enum : Outport  Port=9
  VINP_RrMCU3SWVer_enum : Outport  Port=10
  VINP_RrMCUTempWarn_enum : Outport  Port=11
  VINP_RrTMTempWarn_enum : Outport  Port=12
  wires:
  BHAL_outputs/1 -> [BHAL_outputs]
  inp_CanValid_bus/1 -> [inp_CanValid_bus]
  [BHAL_outputs] -> slr_VHAL_MCUBRLLCTempWarnSta_enum/1
  slr_VHAL_MCUBRLLCTempWarnSta_enum/1 -> MCUBRLLCTempWarnSta/1  "<VHAL_MCUBRLLCTempWarnSta_enum>"
  True_VHAL_MCUBRLLCTempWarnSta_enum/1 -> MCUBRLLCTempWarnSta/2
  [inp_CanValid_bus] -> slr1_1/1
  slr1_1/1 -> MCUBRLLCTempWarnSta/3  "<VINP_CANMsgValidMCUBR2_flg>"
  MCUBRLLCTempWarnSta/1 -> VINP_MCUBRLLCTempWarnSta_enum/1  "VINP_MCUBRLLCTempWarnSta_enum"
  MCUBRLLCTempWarnSta/2 -> Terminator_1/1
  [BHAL_outputs] -> slr_VHAL_RrCoolanttempReq_cnt/1
  slr_VHAL_RrCoolanttempReq_cnt/1 -> RrCoolanttempReq/1  "<VHAL_RrCoolanttempReq_cnt>"
  True_VHAL_RrCoolanttempReq_cnt/1 -> RrCoolanttempReq/2
  [inp_CanValid_bus] -> slr1_2/1
  slr1_2/1 -> RrCoolanttempReq/3  "<VINP_CANMsgValidMCUBR2_flg>"
  RrCoolanttempReq/1 -> VINP_RrCoolanttempReq_cnt/1  "VINP_RrCoolanttempReq_cnt"
  RrCoolanttempReq/2 -> Terminator_2/1
  [BHAL_outputs] -> slr_VHAL_RrFailcode1_enum/1
  slr_VHAL_RrFailcode1_enum/1 -> RrFailcode1/1  "<VHAL_RrFailcode1_enum>"
  True_VHAL_RrFailcode1_enum/1 -> RrFailcode1/2
  [inp_CanValid_bus] -> slr1_3/1
  slr1_3/1 -> RrFailcode1/3  "<VINP_CANMsgValidMCUBR2_flg>"
  RrFailcode1/1 -> VINP_RrFailcode1_enum/1  "VINP_RrFailcode1_enum"
  RrFailcode1/2 -> Terminator_3/1
  [BHAL_outputs] -> slr_VHAL_RrFailcode2_enum/1
  slr_VHAL_RrFailcode2_enum/1 -> RrFailcode2/1  "<VHAL_RrFailcode2_enum>"
  True_VHAL_RrFailcode2_enum/1 -> RrFailcode2/2
  [inp_CanValid_bus] -> slr1_4/1
  slr1_4/1 -> RrFailcode2/3  "<VINP_CANMsgValidMCUBR2_flg>"
  RrFailcode2/1 -> VINP_RrFailcode2_enum/1  "VINP_RrFailcode2_enum"
  RrFailcode2/2 -> Terminator_4/1
  [BHAL_outputs] -> slr_VHAL_RrFailcodehistory1_enum/1
  slr_VHAL_RrFailcodehistory1_enum/1 -> RrFailcodehistory1/1  "<VHAL_RrFailcodehistory1_enum>"
  True_VHAL_RrFailcodehistory1_enum/1 -> RrFailcodehistory1/2
  [inp_CanValid_bus] -> slr1_5/1
  slr1_5/1 -> RrFailcodehistory1/3  "<VINP_CANMsgValidMCUBR2_flg>"
  RrFailcodehistory1/1 -> VINP_RrFailcodehistory1_enum/1  "VINP_RrFailcodehistory1_enum"
  RrFailcodehistory1/2 -> Terminator_5/1
  [BHAL_outputs] -> slr_VHAL_RrFailcodehistory2_enum/1
  slr_VHAL_RrFailcodehistory2_enum/1 -> RrFailcodehistory2/1  "<VHAL_RrFailcodehistory2_enum>"
  True_VHAL_RrFailcodehistory2_enum/1 -> RrFailcodehistory2/2
  [inp_CanValid_bus] -> slr1_6/1
  slr1_6/1 -> RrFailcodehistory2/3  "<VINP_CANMsgValidMCUBR2_flg>"
  RrFailcodehistory2/1 -> VINP_RrFailcodehistory2_enum/1  "VINP_RrFailcodehistory2_enum"
  RrFailcodehistory2/2 -> Terminator_6/1
  [BHAL_outputs] -> slr_VHAL_RrLLCTemp_C/1
  slr_VHAL_RrLLCTemp_C/1 -> RrLLCTemp/1  "<VHAL_RrLLCTemp_C>"
  True_VHAL_RrLLCTemp_C/1 -> RrLLCTemp/2
  [inp_CanValid_bus] -> slr1_7/1
  slr1_7/1 -> RrLLCTemp/3  "<VINP_CANMsgValidMCUBR2_flg>"
  RrLLCTemp/1 -> VINP_RrLLCTemp_C/1  "VINP_RrLLCTemp_C"
  RrLLCTemp/2 -> Terminator_7/1
  [BHAL_outputs] -> slr_VHAL_RrLLCflowReq_Lpmin/1
  slr_VHAL_RrLLCflowReq_Lpmin/1 -> RrLLCflowReq/1  "<VHAL_RrLLCflowReq_Lpmin>"
  True_VHAL_RrLLCflowReq_Lpmin/1 -> RrLLCflowReq/2
  [inp_CanValid_bus] -> slr1_8/1
  slr1_8/1 -> RrLLCflowReq/3  "<VINP_CANMsgValidMCUBR2_flg>"
  RrLLCflowReq/1 -> VINP_RrLLCflowReq_Lpmin/1  "VINP_RrLLCflowReq_Lpmin"
  RrLLCflowReq/2 -> Terminator_8/1
  [BHAL_outputs] -> slr_VHAL_RrMCU3HWVer_enum/1
  slr_VHAL_RrMCU3HWVer_enum/1 -> RrMCU3HWVer/1  "<VHAL_RrMCU3HWVer_enum>"
  True_VHAL_RrMCU3HWVer_enum/1 -> RrMCU3HWVer/2
  [inp_CanValid_bus] -> slr1_9/1
  slr1_9/1 -> RrMCU3HWVer/3  "<VINP_CANMsgValidMCUBR2_flg>"
  RrMCU3HWVer/1 -> VINP_RrMCU3HWVer_enum/1  "VINP_RrMCU3HWVer_enum"
  RrMCU3HWVer/2 -> Terminator_9/1
  [BHAL_outputs] -> slr_VHAL_RrMCU3SWVer_enum/1
  slr_VHAL_RrMCU3SWVer_enum/1 -> RrMCU3SWVer/1  "<VHAL_RrMCU3SWVer_enum>"
  True_VHAL_RrMCU3SWVer_enum/1 -> RrMCU3SWVer/2
  [inp_CanValid_bus] -> slr1_10/1
  slr1_10/1 -> RrMCU3SWVer/3  "<VINP_CANMsgValidMCUBR2_flg>"
  RrMCU3SWVer/1 -> VINP_RrMCU3SWVer_enum/1  "VINP_RrMCU3SWVer_enum"
  RrMCU3SWVer/2 -> Terminator_10/1
  [BHAL_outputs] -> slr_VHAL_RrMCUTempWarn_enum/1
  slr_VHAL_RrMCUTempWarn_enum/1 -> RrMCUTempWarn/1  "<VHAL_RrMCUTempWarn_enum>"
  True_VHAL_RrMCUTempWarn_enum/1 -> RrMCUTempWarn/2
  [inp_CanValid_bus] -> slr1_11/1
  slr1_11/1 -> RrMCUTempWarn/3  "<VINP_CANMsgValidMCUBR2_flg>"
  RrMCUTempWarn/1 -> VINP_RrMCUTempWarn_enum/1  "VINP_RrMCUTempWarn_enum"
  RrMCUTempWarn/2 -> Terminator_11/1
  [BHAL_outputs] -> slr_VHAL_RrTMTempWarn_enum/1
  slr_VHAL_RrTMTempWarn_enum/1 -> RrTMTempWarn/1  "<VHAL_RrTMTempWarn_enum>"
  True_VHAL_RrTMTempWarn_enum/1 -> RrTMTempWarn/2
  [inp_CanValid_bus] -> slr1_12/1
  slr1_12/1 -> RrTMTempWarn/3  "<VINP_CANMsgValidMCUBR2_flg>"
  RrTMTempWarn/1 -> VINP_RrTMTempWarn_enum/1  "VINP_RrTMTempWarn_enum"
  RrTMTempWarn/2 -> Terminator_12/1
